simulink library "pouchPackExample"  (R2024b)
settings: Solver=VariableStepAuto  StartTime=0.0  StopTime=10.0  RelTol=1e-3
undefined symbols (not defined in the file or in its folder): battery_builder_rtmsupport, gcbh
libraries: nesl_utility x3, batt_lib x2, pouchPackExample_lib x1
settings Model: Creator=xiangchz  LastModifiedBy=xiangchz

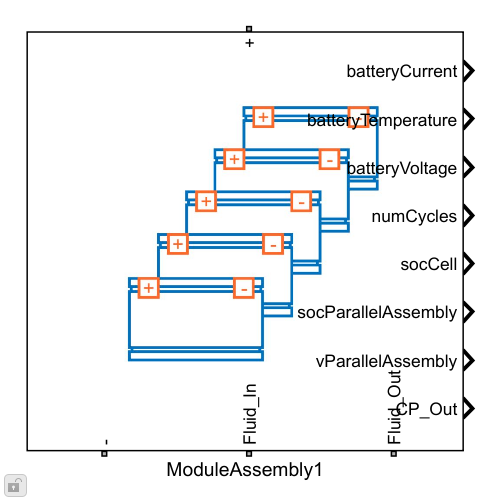
[thumbnail: Simulink's stored preview of the top-level diagram]
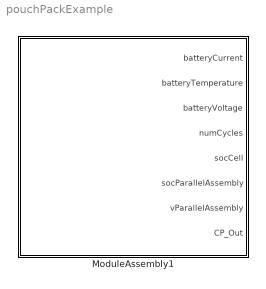
== system pouchPackExample ==
  ModuleAssembly1 : Subsystem  LoadFcn=battery_builder_rtmsupport('loadfcn',gcbh);
      settings: CopyFcn=battery_builder_rtmsupport('copyfcn',gcbh);  PreCopyFcn=battery_builder_rtmsupport('precopyfcn',gcbh);  PreDeleteFcn=battery_builder_rtmsupport('predeletefcn',gcbh);  PortSchema="{\"entries\":[{\"content\":{\"sides\":[{\"content\":{\"connectorIds\":[\"LConn1\"]},\"type\":\"ConnectorPlacement.EquallySpacedRectSide\",\"uuid\":\"5b9bd66e-6eb4-47f7-a339-4edb451c37cc\"},{\"content\":{\"connectorIds\":[\"RConn1\",\"RConn2\",\"RConn3\"],\"side\":\"RIGHT\"},\"type\":\"ConnectorPlacement.EquallySpacedRectSide\",\"uuid\":\"4e53519a-4f95-4811-a8d7-c955c8344f39\"},{\"content\":{\"side\":\"TOP\"},\"type\":\"ConnectorPlacement.EquallySpacedRectSide\",\"uuid\":\"854d433f-9843-4a4d-81aa-2c94c8c627b5\"},{\"content\":{\"connectorIds\":[\"Out1\",\"Out2\",\"Out3\",\"Out4\",\"Out5\",\"Out6\",\"Out7\",\"Out8\"],\"side\":\"BOTTOM\"},\"type\":\"ConnectorPlacement.EquallySpacedRectSide\",\"uuid\":\"6bf6c765-41ee-4c73-bb70-45bb729858cc\"}]},\"type\":\"ConnectorPlacement.EquallySpacedConnector\",\"uuid\":\"d3ba8235-896f-47d4-808e-c28edfccefd3\"}],\"packageUris\":[\"http://schema.mathworks.com/mf0/Connector/R2020b\"],\"version\":\"1.0\"}"
      mask Display: image('$imagefile')

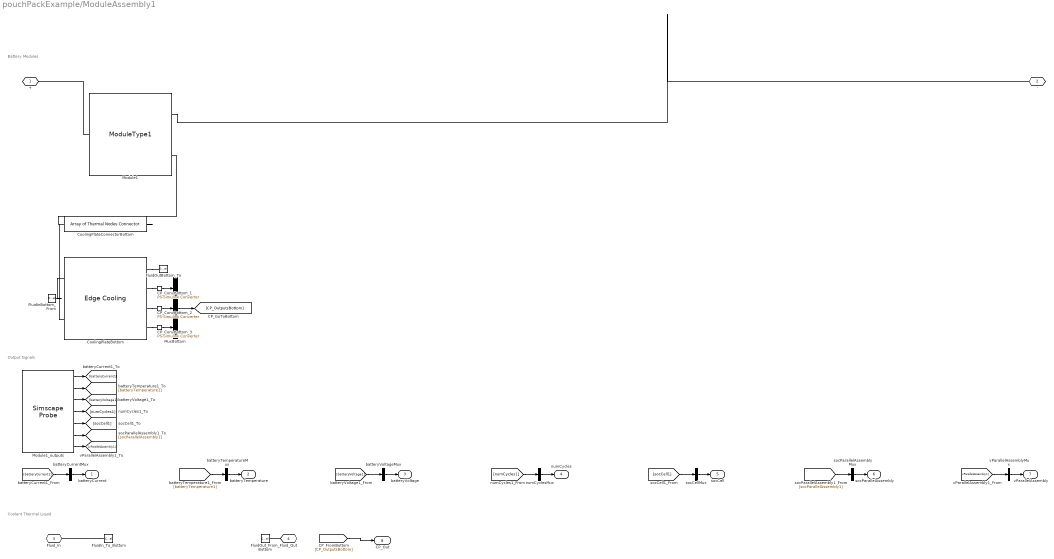
== system pouchPackExample/ModuleAssembly1 ==
  note: Battery Modules
  note: Output Signals
  note: Coolant Thermal Liquid
  CP_ConvBottom_1 : nesl_utility/PS-Simulink Converter  PhysicalDomain=network_engine_domain  SubClassName=ps_output  LeftPortType=input  RightPortType=output  PseudoPeriodic=off  Frequencies=[]  VectorFormat=inherit  Unit=inherit  AffineConversion=off
  CP_ConvBottom_2 : nesl_utility/PS-Simulink Converter  PhysicalDomain=network_engine_domain  SubClassName=ps_output  LeftPortType=input  RightPortType=output  PseudoPeriodic=off  Frequencies=[]  VectorFormat=inherit  Unit=inherit  AffineConversion=off
  CP_ConvBottom_3 : nesl_utility/PS-Simulink Converter  PhysicalDomain=network_engine_domain  SubClassName=ps_output  LeftPortType=input  RightPortType=output  PseudoPeriodic=off  Frequencies=[]  VectorFormat=inherit  Unit=inherit  AffineConversion=off
  CoolingPlateBottom : batt_lib/Thermal/Edge Cooling  plateConnectivity=simscape.battery.enum.thermal.coolingPlateConnectivity.singleSided  numBattThermalNodes1=CoolingPlateBottom.numBattThermalNodes1  dimensionThermalNodes1=CoolingPlateBottom.dimensionThermalNodes1  locationThermalNodes1=CoolingPlateBottom.locationThermalNodes1  numBattThermalNodes2=1  dimensionThermalNodes2=ones(1, 2)  locationThermalNodes2=ones(1, 2)  plateDimX=CoolingPlateBottom.plateDimX  plateDimY=CoolingPlateBottom.plateDimY  plateTh=CoolingPlateBottom.plateTh m  plateThCond=CoolingPlateBottom.plateThCond W/(K*m)  plateDen=CoolingPlateBottom.plateDen kg/m^3  plateCp=CoolingPlateBottom.plateCp J/(K*kg)  plateTemp_ini=CoolingPlateBottom.plateTemp_ini K  Re_lam=CoolingPlateBottom.Re_lam  Re_tur=CoolingPlateBottom.Re_tur  Nu_lam=CoolingPlateBottom.Nu_lam  length_add=CoolingPlateBottom.length_add m  shape_factor=CoolingPlateBottom.shape_factor  selectEdgeOrientation=simscape.battery.enum.thermal.coolingEdgeDirection.alongX0  channelDia=CoolingPlateBottom.channelDia m  channelArea=CoolingPlateBottom.channelArea m^2  roughnessPipe=CoolingPlateBottom.roughnessPipe m
      settings: InternalSimscapePortConfiguration="{\"Bottom\":[],\"Left\":[{\"id\":\"fluid_in\",\"label\":\"fluid_in\",\"type\":\"foundation.thermal_liquid.thermal_liquid\"}],\"Right\":[{\"id\":\"fluid_out\",\"label\":\"fluid_out\",\"type\":\"foundation.thermal_liquid.thermal_liquid\"},{\"id\":\"plotPlateT\",\"label\":\"Tp\",\"type\":\"output\"},{\"id\":\"tempSensor\",\"label\":\"dT\",\"type\":\"output\"},{\"id\":\"presSensor\",\"label\":\"dP\",\"type\":\"output\"}],\"Top\":[{\"id\":\"Side1\",\"label\":\"Surf1\",\"type\":\"foundation.thermal.thermal\"}]}"
  CoolingPlateConnectorBottom : batt_lib/Thermal/Array of Thermal Nodes Connector  numInputConnections=1  concatenateDimension=2  complementaryDimensionsSize=1  inNode1NumElements=3  inNode2NumElements=1  inNode3NumElements=1  inNode4NumElements=1  inNode5NumElements=1  inNode6NumElements=1  inNode7NumElements=1  inNode8NumElements=1  inNode9NumElements=1  inNode10NumElements=1  inNode11NumElements=1  inNode12NumElements=1  inNode13NumElements=1  inNode14NumElements=1  inNode15NumElements=1  inNode16NumElements=1  inNode17NumElements=1  inNode18NumElements=1  inNode19NumElements=1  inNode20NumElements=1  inNode21NumElements=1  inNode22NumElements=1  inNode23NumElements=1  inNode24NumElements=1  inNode25NumElements=1  inNode26NumElements=1  inNode27NumElements=1  inNode28NumElements=1  inNode29NumElements=1  inNode30NumElements=1  inNode31NumElements=1  inNode32NumElements=1  inNode33NumElements=1  inNode34NumElements=1  inNode35NumElements=1  inNode36NumElements=1  inNode37NumElements=1  inNode38NumElements=1  inNode39NumElements=1  inNode40NumElements=1  inNode41NumElements=1  inNode42NumElements=1  inNode43NumElements=1  inNode44NumElements=1  inNode45NumElements=1  inNode46NumElements=1  inNode47NumElements=1  inNode48NumElements=1  inNode49NumElements=1  inNode50NumElements=1
      settings: InternalSimscapePortConfiguration="{\"Bottom\":[{\"id\":\"outConn\",\"label\":\"outConn\",\"type\":\"foundation.thermal.thermal\"}],\"Left\":[],\"Right\":[],\"Top\":[{\"id\":\"inConn1\",\"label\":\"inConn1\",\"type\":\"foundation.thermal.thermal\"}]}"
  FluidInBottom_From : ConnectionLabel  Label=FluidIn_To_Bottom
  FluidIn_To_Bottom : ConnectionLabel  Label=FluidIn_To_Bottom
  FluidOutBottom_To : ConnectionLabel  Label=FluidOut_From_Bottom
  FluidOut_From_Bottom : ConnectionLabel  Label=FluidOut_From_Bottom
  Module1 : pouchPackExample_lib/Modules/ModuleType1  BatteryCapacityCell=ModuleType1.BatteryCapacityCell A*hr  ExtrapolationMethodCell=simscape.enum.extrapolation.nearest  SOCBreakpointsCell=ModuleType1.SOCBreakpointsCell  TemperatureBreakpointsCell=ModuleType1.TemperatureBreakpointsCell K  OpenCircuitVoltageThermalCell=ModuleType1.OpenCircuitVoltageThermalCell V  VoltageRangeCell=ModuleType1.VoltageRangeCell V  ResistanceSOCBreakpointsCell=ModuleType1.ResistanceSOCBreakpointsCell  ResistanceTemperatureBreakpointsCell=ModuleType1.ResistanceTemperatureBreakpointsCell K  R0ThermalCell=ModuleType1.R0ThermalCell Ohm  R1ThermalCell=ModuleType1.R1ThermalCell Ohm  Tau1ThermalCell=ModuleType1.Tau1ThermalCell s  BatteryThermalMassCell=ModuleType1.BatteryThermalMassCell J/K  CoolantResistance=ModuleType1.CoolantResistance K/W  P=4  S=14  SeriesGrouping=[4, 5, 5]  ParallelGrouping=[1, 1, 1]  socCell_specify=on  socCell_priority=High  socCell=Module1.socCell  socCell_nominal_specify=off  socCell_nominal_value=1  socCell_nominal_unit=1  numCycles_specify=on  numCycles_priority=High  numCycles=Module1.numCycles  numCycles_nominal_specify=off  numCycles_nominal_value=1  numCycles_nominal_unit=1  batteryVoltage_specify=on  batteryVoltage_priority=None  batteryVoltage=Module1.batteryVoltage V  batteryVoltage_nominal_specify=off  batteryVoltage_nominal_value=1  batteryVoltage_nominal_unit=V  batteryCurrent_specify=on  batteryCurrent_priority=None  batteryCurrent=Module1.batteryCurrent A  batteryCurrent_nominal_specify=off  batteryCurrent_nominal_value=1  batteryCurrent_nominal_unit=A  batteryTemperature_specify=on  batteryTemperature_priority=High  batteryTemperature=Module1.batteryTemperature K  batteryTemperature_nominal_specify=off  batteryTemperature_nominal_value=1  batteryTemperature_nominal_unit=K  vParallelAssembly_specify=on  vParallelAssembly_priority=None  vParallelAssembly=Module1.vParallelAssembly V  vParallelAssembly_nominal_specify=off  vParallelAssembly_nominal_value=1  vParallelAssembly_nominal_unit=V  socParallelAssembly_specify=on  socParallelAssembly_priority=None  socParallelAssembly=Module1.socParallelAssembly  socParallelAssembly_nominal_specify=off  socParallelAssembly_nominal_value=1  socParallelAssembly_nominal_unit=1
      settings: InternalSimscapePortConfiguration="{\"Bottom\":[{\"id\":\"n\",\"label\":\"-\",\"type\":\"foundation.electrical.electrical\"},{\"id\":\"BottomExtClnt\",\"label\":\"CPB\",\"type\":\"foundation.thermal.thermal\"}],\"Left\":[],\"Right\":[],\"Top\":[{\"id\":\"p\",\"label\":\"+\",\"type\":\"foundation.electrical.electrical\"}]}"
  Module1_outputs : SimscapeProbe  BoundBlock=2  Variables="{\"batteryCurrent\":{\"Unit\":\"A\",\"PortLabel\":\"batteryCurrent\",\"Probing\":\"ON\"},\"batteryTemperature\":{\"Unit\":\"K\",\"PortLabel\":\"batteryTemperature\",\"Probing\":\"ON\"},\"batteryVoltage\":{\"Unit\":\"V\",\"PortLabel\":\"batteryVoltage\",\"Probing\":\"ON\"},\"numCycles\":{\"Unit\":\"1\",\"PortLabel\":\"numCycles\",\"Probing\":\"ON\"},\"socCell\":{\"Unit\":\"1\",\"PortLabel\":\"socCell\",\"Probing\":\"ON\"},\"socParallelAssembly\":{\"Unit\":\"1\",\"PortLabel\":\"socParallelAssembly\",\"Probing\":\"ON\"},\"vParallelAssembly\":{\"Unit\":\"V\",\"PortLabel\":\"vParallelAssembly\",\"Probing\":\"ON\"}}"
  MuxBottom : Mux  Inputs=3
  batteryCurrentMux : Mux  Inputs=1
  batteryTemperatureMux : Mux  Inputs=1
  batteryVoltageMux : Mux  Inputs=1
  numCyclesMux : Mux  Inputs=1
  socCellMux : Mux  Inputs=1
  socParallelAssemblyMux : Mux  Inputs=1
  vParallelAssemblyMux : Mux  Inputs=1
  + : PMIOPort  Side=Left
  - : PMIOPort  Port=2  Side=Right
  Fluid_In : PMIOPort  Port=3  Side=Right  ConnectionType=Connection: foundation.thermal_liquid.thermal_liquid
  Fluid_Out : PMIOPort  Port=4  Side=Right  ConnectionType=Connection: foundation.thermal_liquid.thermal_liquid
  batteryCurrent : Outport
  batteryTemperature : Outport  Port=2
  batteryVoltage : Outport  Port=3
  numCycles : Outport  Port=4
  socCell : Outport  Port=5
  socParallelAssembly : Outport  Port=6
  vParallelAssembly : Outport  Port=7
  CP_Out : Outport  Port=8
  wires:
  Module1_outputs/1 -> [batteryCurrent1]
  batteryCurrentMux/1 -> batteryCurrent/1
  [batteryCurrent1] -> batteryCurrentMux/1
  Module1_outputs/2 -> [batteryTemperature1]
  batteryTemperatureMux/1 -> batteryTemperature/1
  [batteryTemperature1] -> batteryTemperatureMux/1
  Module1_outputs/3 -> [batteryVoltage1]
  batteryVoltageMux/1 -> batteryVoltage/1
  [batteryVoltage1] -> batteryVoltageMux/1
  Module1_outputs/4 -> [numCycles1]
  numCyclesMux/1 -> numCycles/1
  [numCycles1] -> numCyclesMux/1
  Module1_outputs/5 -> [socCell1]
  socCellMux/1 -> socCell/1
  [socCell1] -> socCellMux/1
  Module1_outputs/6 -> [socParallelAssembly1]
  socParallelAssemblyMux/1 -> socParallelAssembly/1
  [socParallelAssembly1] -> socParallelAssemblyMux/1
  Module1_outputs/7 -> [vParallelAssembly1]
  vParallelAssemblyMux/1 -> vParallelAssembly/1
  [vParallelAssembly1] -> vParallelAssemblyMux/1
  CP_ConvBottom_1/1 -> MuxBottom/1
  CP_ConvBottom_2/1 -> MuxBottom/2
  CP_ConvBottom_3/1 -> MuxBottom/3
  MuxBottom/1 -> [CP_OutputsBottom]
  [CP_OutputsBottom] -> CP_Out/1
  connections:
  Module1/LConn1 -- +/RConn1
  Module1/RConn1 -- -/RConn1
  CoolingPlateConnectorBottom/LConn1 -- Module1/RConn2
  CoolingPlateConnectorBottom/RConn1 -- CoolingPlateBottom/LConn2
  FluidIn_To_Bottom/LConn1 -- Fluid_In/RConn1
  Fluid_Out/RConn1 -- FluidOut_From_Bottom/LConn1
  FluidInBottom_From/LConn1 -- CoolingPlateBottom/LConn1
  CoolingPlateBottom/RConn1 -- FluidOutBottom_To/LConn1
  CoolingPlateBottom/RConn2 -- CP_ConvBottom_1/LConn1
  CoolingPlateBottom/RConn3 -- CP_ConvBottom_2/LConn1
  CoolingPlateBottom/RConn4 -- CP_ConvBottom_3/LConn1
